simulink model "TBRe19_ECU_Torque_request_TSS_ON"  (R2017b)
settings: Solver=FixedStepDiscrete  StartTime=0.0  StopTime=inf  FixedStep=0.0001  RelTol=1e-3
PostLoadFcn:
  | model_init();
libraries: simulink x17
(part 4 of 6)

== system TBRe19_ECU_Torque_request_TSS_ON/MainTask/Pre_Processing_Layer/Pedal_Box ==
  note: Throttle 20 and Brake 10 are arbitrary values (not rules)
  note: Overall Functionality:
      | - All pedal box sensor values are checked to ensure that they are in the correct voltage range
      | - These sensors are then scaled to be between 0-100 %
      | - APPS Implausibility is performed
      | - Brake pedal implausibility is performed
      | - Thresholds for when brake is considered active, and throttle is considered active are set here (used for RTD and Brake Light activation respectively)
  DAL_In : Inport
  APPS and BP Plausibility : Subsystem
  APPS_Implausibility_Check : Subsystem
  BPPS_Implausibility_Check : Subsystem
  Bus Creator : BusCreator  Inputs=12
  Bus Selector : BusSelector  OutputSignals=DAL_Hardwired.Throttle1_Voltage,DAL_Hardwired.Throttle2_Voltage,DAL_Hardwired.Brake_POT,DAL_Hardwired.Brake1_Pressure,DAL_Hardwired.Brake2_Pressure
  Memory read : S-Function  FunctionName=NsiMem_Read  Parameters=name_var,type_var,size_var,tunable_var  SFunctionDeploymentMode=off  EnableBusSupport=off  mask(Memory read){name_var=Throttle_Active_Threshold, type_var=Unsigned Byte, size_var=1, tunable_var=on}
      mask prompts: name_var "Variable name :"; type_var "Type :"; size_var "Dim of table :"; tunable_var "Is Tunable By USB?"
      mask help: Reads current value of variable memory declared in the configurator block in calibration page.
      mask init:
      | NsiMem_Read_InitializationFcn();
      settings: OpenFcn=NsiMem_Read_OpenFcn();
      mask Help:
      | eval('block=get_param(gcb, ''RTWdata'');')
      | web([docroot '\toolbox\MUXlink\html\blocks/' block.MUXlink_BlockType '.html'])
      mask TypeOptions name_var: Gearing_Ratio | Wheel_Size | Brake1_High | Brake2_High | Throttle1_High | Throttle2_High | Brake1_Low | Brake2_Low | Throttle1_Low | Throttle2_Low | Max_Torque_Std | Max_Torque_Boost | MCU_Ignition | LV_Low_Voltage_Warning | MCUMotor_Temp_Warning | Target_Slip_Ratio | TC_P_Gain | MinTC_Torque | Max_Regen | Throttle_Active_Threshold | Brake_Active_Threshold | INV_Torque_limit | INV_Speed_Limit_Fwd | INV_Speed_limit_Rev | INV_DC_Link_Target | INV_DC_Link_Regen_Imax | INV_DC_Link_Discharge_Imax | INV_Regen_Torque_Limit | INV_Id_Debug | INV_Iq_debug
      mask Callback name_var: NsiMem_Read_ApplyFcn(1);
      mask TypeOptions type_var: Boolean | Signed Byte | Unsigned Byte | Signed Word | Unsigned Word | Signed Double Word | Unsigned Double Word | Single Float | Double Float
      mask Callback type_var: NsiMem_Read_ApplyFcn(2);
      mask Callback size_var: NsiMem_Read_ApplyFcn(3);
      mask Callback tunable_var: NsiMem_Read_ApplyFcn(4);
      mask Display: image(imread('nsi.bmp'));text(0.5, 0.35, 'Throttle_Active_Threshold', 'horizontalAlignment', 'center', 'verticalAlignment', 'base');plot([0.05 0.05 0.05 0.05 0.05 0.05 0.05 0.05 0.05 0.05]);port_label('output', 1, 'Read');
  Memory read1 : S-Function  FunctionName=NsiMem_Read  Parameters=name_var,type_var,size_var,tunable_var  SFunctionDeploymentMode=off  EnableBusSupport=off  mask(Memory read){name_var=Brake_Active_Threshold, type_var=Unsigned Byte, size_var=1, tunable_var=on}
      mask prompts: name_var "Variable name :"; type_var "Type :"; size_var "Dim of table :"; tunable_var "Is Tunable By USB?"
      mask help: Reads current value of variable memory declared in the configurator block in calibration page.
      mask init:
      | NsiMem_Read_InitializationFcn();
      settings: OpenFcn=NsiMem_Read_OpenFcn();
      mask Help:
      | eval('block=get_param(gcb, ''RTWdata'');')
      | web([docroot '\toolbox\MUXlink\html\blocks/' block.MUXlink_BlockType '.html'])
      mask TypeOptions name_var: Gearing_Ratio | Wheel_Size | Brake1_High | Brake2_High | Throttle1_High | Throttle2_High | Brake1_Low | Brake2_Low | Throttle1_Low | Throttle2_Low | Max_Torque_Std | Max_Torque_Boost | MCU_Ignition | LV_Low_Voltage_Warning | MCUMotor_Temp_Warning | Target_Slip_Ratio | TC_P_Gain | MinTC_Torque | Max_Regen | Throttle_Active_Threshold | Brake_Active_Threshold | INV_Torque_limit | INV_Speed_Limit_Fwd | INV_Speed_limit_Rev | INV_DC_Link_Target | INV_DC_Link_Regen_Imax | INV_DC_Link_Discharge_Imax | INV_Regen_Torque_Limit | INV_Id_Debug | INV_Iq_debug
      mask Callback name_var: NsiMem_Read_ApplyFcn(1);
      mask TypeOptions type_var: Boolean | Signed Byte | Unsigned Byte | Signed Word | Unsigned Word | Signed Double Word | Unsigned Double Word | Single Float | Double Float
      mask Callback type_var: NsiMem_Read_ApplyFcn(2);
      mask Callback size_var: NsiMem_Read_ApplyFcn(3);
      mask Callback tunable_var: NsiMem_Read_ApplyFcn(4);
      mask Display: image(imread('nsi.bmp'));text(0.5, 0.35, 'Brake_Active_Threshold', 'horizontalAlignment', 'center', 'verticalAlignment', 'base');plot([0.05 0.05 0.05 0.05 0.05 0.05 0.05 0.05 0.05 0.05]);port_label('output', 1, 'Read');
  Relational Operator : RelationalOperator  OutDataTypeStr=boolean  RndMeth=Simplest
  Relational Operator1 : RelationalOperator  OutDataTypeStr=boolean  RndMeth=Simplest
  Sensor Plausibility : Subsystem
  Terminator : Terminator
  UsbTx1 : S-Function  FunctionName=NsiUsb_Tx  Parameters=signame,resolution,offset,unite  SFunctionDeploymentMode=off  EnableBusSupport=off  mask(MUXlink Usb Tx){signame=Throttle_merge, resolution=1, offset=0, unite=%}
      mask prompts: signame "Signal name ?"; resolution "Resolution ?"; offset "Offset ?"; unite "Unit ?"
      mask help: Transmit a frame on the USB Channel.
      mask init:
      | NsiUsb_Tx_InitializationFcn();
      settings: OpenFcn=NsiUsb_Tx_OpenFcn();
      mask Help:
      | eval('block=get_param(gcb, ''RTWdata'');')
      | web([docroot '\toolbox\MUXlink\html\blocks/' block.MUXlink_BlockType '.html'])
      mask Callback signame: NsiUsb_Tx_ApplyFcn(1);
      mask Callback resolution: NsiUsb_Tx_ApplyFcn(2);
      mask Callback offset: NsiUsb_Tx_ApplyFcn(3);
      mask Callback unite: NsiUsb_Tx_ApplyFcn(4);
      mask Display: image(imread('nsi.bmp'));text(0.5, 0.2, 'USB Tx', 'horizontalAlignment', 'center', 'verticalAlignment', 'base');plot([0.05 0.05 0.05 0.05 0.05 0.05 0.05 0.05 0.05 0.05]);port_label('input',1, 'Throttle_merge');
  Voltage_to_% Conversion : Subsystem
  Pedal_Box_Data : Outport
  wires:
  Bus Creator/1 -> Pedal_Box_Data/1
  DAL_In/1 -> Bus Selector/1
  Voltage_to_% Conversion/1(T1%) -> Bus Creator/2, APPS_Implausibility_Check/1(Throttle1_Per)  "Throttle1_Per"
  Voltage_to_% Conversion/2(T2%) -> Bus Creator/3, APPS_Implausibility_Check/2(Throttle2_Per)  "Throttle2_Per"
  Relational Operator1/1 -> Bus Creator/6  "Throttle_Bool"
  Relational Operator/1 -> Bus Creator/8  "Brake_Bool"
  APPS and BP Plausibility/1(Throttle_%) -> Relational Operator1/1, UsbTx1/1, Bus Creator/5  "Throttle_Percentage"
  APPS and BP Plausibility/2(APPS_BP_Implausibility) -> Bus Creator/7  "APPS_BP_Implausibility"
  APPS_Implausibility_Check/1(APPS_Implausibility) -> Bus Creator/4  "APPS_Implausibility"
  APPS_Implausibility_Check/2(Throttle_%) -> APPS and BP Plausibility/1(Throttle_In)
  Sensor Plausibility/1(Pedal_Sensor_Fail) -> Bus Creator/1  "Pedal_Sensor_Fail"
  Bus Selector/1 -> Sensor Plausibility/1(<Throttle1_Voltage>)  "<Throttle1_Voltage>"
  Bus Selector/2 -> Sensor Plausibility/2(<Throttle2_Voltage>)  "<Throttle2_Voltage>"
  Bus Selector/3 -> Sensor Plausibility/3(<Brake_Voltage>)  "<Brake_POT>"
  Sensor Plausibility/2(TV1_Out) -> Voltage_to_% Conversion/1(Throttle1)
  Sensor Plausibility/3(TV2_Out) -> Voltage_to_% Conversion/2(Throttle2)
  Sensor Plausibility/4(BVPot_Out) -> Voltage_to_% Conversion/3(BrakePOT)
  Bus Selector/4 -> Sensor Plausibility/4(<Brake_Voltage>1)  "<Brake1_Pressure>"
  Bus Selector/5 -> Sensor Plausibility/5(<Brake_Voltage>2)  "<Brake2_Pressure>"
  Sensor Plausibility/5(BV1_Out) -> Voltage_to_% Conversion/4(BrakePress1)
  Sensor Plausibility/6(BV1_Out1) -> Voltage_to_% Conversion/5(BrakePress2)
  BPPS_Implausibility_Check/1(Brake_%) -> Relational Operator/1, Bus Creator/9, APPS and BP Plausibility/2(Brake_%)  "Brake_Percentage"
  BPPS_Implausibility_Check/2(BPPS_Implausibility) -> Bus Creator/10  "BPPS_Implausibility"
  Voltage_to_% Conversion/4(BPr%1) -> Bus Creator/11, BPPS_Implausibility_Check/1(Brake1_Per)  "Brake1_Per"
  Voltage_to_% Conversion/5(BPr%2) -> Bus Creator/12, BPPS_Implausibility_Check/2(Brake2_Per)  "Brake2_Per"
  Voltage_to_% Conversion/3(BPot%) -> Terminator/1  "Brake_%"
  Memory read1/1 -> Relational Operator/2
  Memory read/1 -> Relational Operator1/2

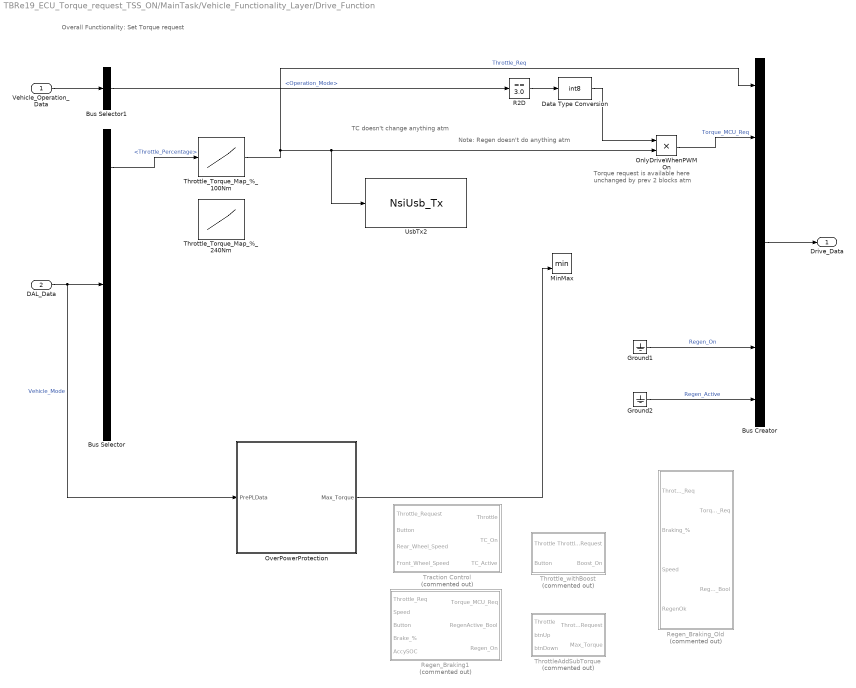
== system TBRe19_ECU_Torque_request_TSS_ON/MainTask/Vehicle_Functionality_Layer/Drive_Function ==
  note: Torque request is available here
      | unchanged by prev 2 blocks atm
  note: TC doesn't change anything atm
  note: Note: Regen doesn't do anything atm
  note: Overall Functionality:
      | Set Torque request
  Vehicle_Operation_Data : Inport
  DAL_Data : Inport  Port=2
  Bus Creator : BusCreator  Inputs=7
  Bus Selector : BusSelector  OutputSignals=Pedal_Box_Data.Throttle_Percentage,DAL_Data.DAL_Hardwired.btnX_Input,DAL_Data.DAL_Hardwired.btnY_Input,DAL_Data.DAL_Hardwired.btnZ_Input
  Bus Selector1 : BusSelector  OutputSignals=Operation_Mode
  Data Type Conversion : DataTypeConversion  OutDataTypeStr=int8
  Ground1 : Ground
  Ground2 : Ground
  MinMax : MinMax  Inputs=2
  OnlyDriveWhenPWMOn : Product  OutDataTypeStr=int16
  OverPowerProtection : Subsystem
  R2D : simulink/Logic and Bit Operations/Compare To Constant  relop===  const=3.0  OutDataTypeStr=boolean
  Regen_Braking1 : Subsystem  Commented=on
  Regen_Braking_Old : Subsystem  Commented=on
  ThrottleAddSubTorque : Subsystem  Commented=on
  Throttle_Torque_Map_%_100Nm : Lookup_n-D  NumberOfTableDimensions=1  BreakpointsForDimension1=[0,25,100]  Table=[0,10,100]  ExtrapMethod=Clip  UseLastTableValue=on  InternalRulePriority=Speed  OutDataTypeStr=int16  RndMeth=Simplest  InputSameDT=on
  Throttle_Torque_Map_%_240Nm : Lookup_n-D  NumberOfTableDimensions=1  BreakpointsForDimension1=[0,25,100]  Table=[0,20,240]  ExtrapMethod=Clip  UseLastTableValue=on  InternalRulePriority=Speed  OutDataTypeStr=int16  RndMeth=Simplest  InputSameDT=on
  Throttle_withBoost : Subsystem  Commented=on
  Traction Control : Subsystem  Commented=on
  UsbTx2 : S-Function  FunctionName=NsiUsb_Tx  Parameters=signame,resolution,offset,unite  SFunctionDeploymentMode=off  EnableBusSupport=off  mask(MUXlink Usb Tx){signame=TorqueRequestInternal, resolution=1, offset=0, unite=Nm}
      mask prompts: signame "Signal name ?"; resolution "Resolution ?"; offset "Offset ?"; unite "Unit ?"
      mask help: Transmit a frame on the USB Channel.
      mask init:
      | NsiUsb_Tx_InitializationFcn();
      settings: OpenFcn=NsiUsb_Tx_OpenFcn();
      mask Help:
      | eval('block=get_param(gcb, ''RTWdata'');')
      | web([docroot '\toolbox\MUXlink\html\blocks/' block.MUXlink_BlockType '.html'])
      mask Callback signame: NsiUsb_Tx_ApplyFcn(1);
      mask Callback resolution: NsiUsb_Tx_ApplyFcn(2);
      mask Callback offset: NsiUsb_Tx_ApplyFcn(3);
      mask Callback unite: NsiUsb_Tx_ApplyFcn(4);
      mask Display: image(imread('nsi.bmp'));text(0.5, 0.2, 'USB Tx', 'horizontalAlignment', 'center', 'verticalAlignment', 'base');plot([0.05 0.05 0.05 0.05 0.05 0.05 0.05 0.05 0.05 0.05]);port_label('input',1, 'TorqueRequestInternal');
  Drive_Data : Outport
  wires:
  Bus Selector1/1 -> R2D/1  "<Operation_Mode>"
  Bus Selector/1 -> Throttle_Torque_Map_%_100Nm/1  "<Throttle_Percentage>"
  R2D/1 -> Data Type Conversion/1
  Vehicle_Operation_Data/1 -> Bus Selector1/1
  DAL_Data/1 -> OverPowerProtection/1(PrePLData), Bus Selector/1  "Vehicle_Mode"
  OnlyDriveWhenPWMOn/1 -> Bus Creator/2  "Torque_MCU_Req"
  Throttle_Torque_Map_%_100Nm/1 -> UsbTx2/1, OnlyDriveWhenPWMOn/2, Bus Creator/1  "Throttle_Req"
  Bus Creator/1 -> Drive_Data/1
  Data Type Conversion/1 -> OnlyDriveWhenPWMOn/1
  Ground1/1 -> Bus Creator/6  "Regen_On"
  OverPowerProtection/1(Max_Torque) -> MinMax/2
  Ground2/1 -> Bus Creator/7  "Regen_Active"

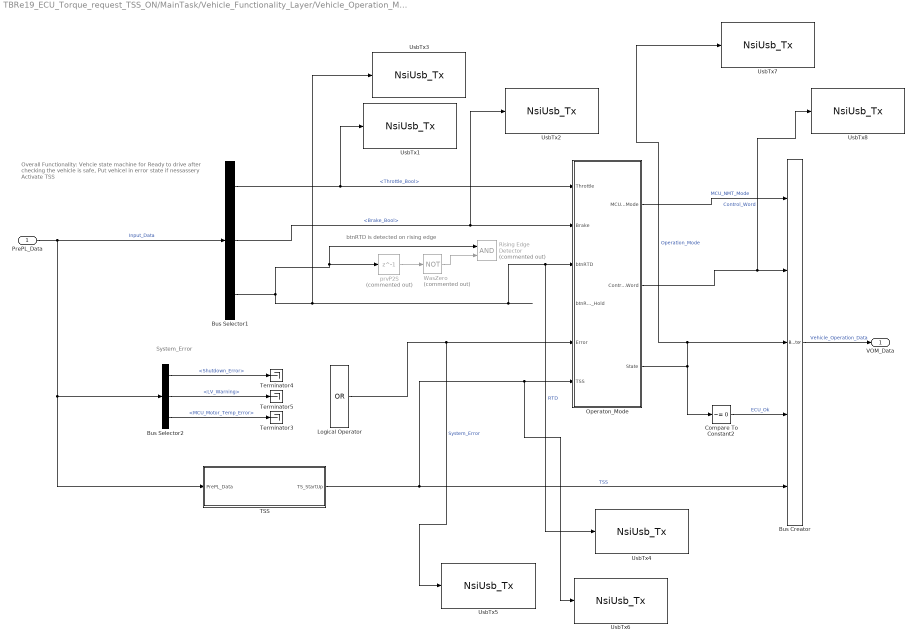
== system TBRe19_ECU_Torque_request_TSS_ON/MainTask/Vehicle_Functionality_Layer/Vehicle_Operation_Mode ==
  note: System_Error
  note: btnRTD is detected on rising edge
  note: Overall Functionality:
      | Vehcie state machine for Ready to drive after checking the vehicle is safe,
      | Put vehicel in error state if nessassery
      | Activate TSS
  PrePL_Data : Inport
  Bus Creator : BusCreator  Inputs=5
  Bus Selector1 : BusSelector  OutputSignals=Pedal_Box_Data.Throttle_Bool,Pedal_Box_Data.Brake_Bool,Buttons.btnRTD
  Bus Selector2 : BusSelector  OutputSignals=DAL_Data.DAL_CAN.DAL_SENSORCAN.Shutdown_Error,LV_Battery.LV_Warning,MCU_Temps_Data.MCU_Motor_Temp_Error
  Compare To Constant2 : simulink/Logic and Bit Operations/Compare To Constant  relop=~=  const=0  OutDataTypeStr=boolean
  Logical Operator : Logic  Operator=OR  Inputs=5  AllPortsSameDT=off  OutDataTypeStr=boolean
  Operaton_Mode : Stateflow chart  TreatAsAtomicUnit=on
  Rising Edge Detector : Logic  Commented=on  AllPortsSameDT=off  OutDataTypeStr=boolean
  TSS : Subsystem
  Terminator3 : Terminator
  Terminator4 : Terminator
  Terminator5 : Terminator
  UsbTx1 : S-Function  FunctionName=NsiUsb_Tx  Parameters=signame,resolution,offset,unite  SFunctionDeploymentMode=off  EnableBusSupport=off  mask(MUXlink Usb Tx){signame=throttle_bool, resolution=1, offset=0, unite=bool}
      mask prompts: signame "Signal name ?"; resolution "Resolution ?"; offset "Offset ?"; unite "Unit ?"
      mask help: Transmit a frame on the USB Channel.
      mask init:
      | NsiUsb_Tx_InitializationFcn();
      settings: OpenFcn=NsiUsb_Tx_OpenFcn();
      mask Help:
      | eval('block=get_param(gcb, ''RTWdata'');')
      | web([docroot '\toolbox\MUXlink\html\blocks/' block.MUXlink_BlockType '.html'])
      mask Callback signame: NsiUsb_Tx_ApplyFcn(1);
      mask Callback resolution: NsiUsb_Tx_ApplyFcn(2);
      mask Callback offset: NsiUsb_Tx_ApplyFcn(3);
      mask Callback unite: NsiUsb_Tx_ApplyFcn(4);
      mask Display: image(imread('nsi.bmp'));text(0.5, 0.2, 'USB Tx', 'horizontalAlignment', 'center', 'verticalAlignment', 'base');plot([0.05 0.05 0.05 0.05 0.05 0.05 0.05 0.05 0.05 0.05]);port_label('input',1, 'throttle_bool');
  UsbTx2 : S-Function  FunctionName=NsiUsb_Tx  Parameters=signame,resolution,offset,unite  SFunctionDeploymentMode=off  EnableBusSupport=off  mask(MUXlink Usb Tx){signame=Brake_bool, resolution=1, offset=0, unite=bool}
      mask prompts: signame "Signal name ?"; resolution "Resolution ?"; offset "Offset ?"; unite "Unit ?"
      mask help: Transmit a frame on the USB Channel.
      mask init:
      | NsiUsb_Tx_InitializationFcn();
      settings: OpenFcn=NsiUsb_Tx_OpenFcn();
      mask Help:
      | eval('block=get_param(gcb, ''RTWdata'');')
      | web([docroot '\toolbox\MUXlink\html\blocks/' block.MUXlink_BlockType '.html'])
      mask Callback signame: NsiUsb_Tx_ApplyFcn(1);
      mask Callback resolution: NsiUsb_Tx_ApplyFcn(2);
      mask Callback offset: NsiUsb_Tx_ApplyFcn(3);
      mask Callback unite: NsiUsb_Tx_ApplyFcn(4);
      mask Display: image(imread('nsi.bmp'));text(0.5, 0.2, 'USB Tx', 'horizontalAlignment', 'center', 'verticalAlignment', 'base');plot([0.05 0.05 0.05 0.05 0.05 0.05 0.05 0.05 0.05 0.05]);port_label('input',1, 'Brake_bool');
  UsbTx3 : S-Function  FunctionName=NsiUsb_Tx  Parameters=signame,resolution,offset,unite  SFunctionDeploymentMode=off  EnableBusSupport=off  mask(MUXlink Usb Tx){signame=rtd_button, resolution=1, offset=0, unite=bool}
      mask prompts: signame "Signal name ?"; resolution "Resolution ?"; offset "Offset ?"; unite "Unit ?"
      mask help: Transmit a frame on the USB Channel.
      mask init:
      | NsiUsb_Tx_InitializationFcn();
      settings: OpenFcn=NsiUsb_Tx_OpenFcn();
      mask Help:
      | eval('block=get_param(gcb, ''RTWdata'');')
      | web([docroot '\toolbox\MUXlink\html\blocks/' block.MUXlink_BlockType '.html'])
      mask Callback signame: NsiUsb_Tx_ApplyFcn(1);
      mask Callback resolution: NsiUsb_Tx_ApplyFcn(2);
      mask Callback offset: NsiUsb_Tx_ApplyFcn(3);
      mask Callback unite: NsiUsb_Tx_ApplyFcn(4);
      mask Display: image(imread('nsi.bmp'));text(0.5, 0.2, 'USB Tx', 'horizontalAlignment', 'center', 'verticalAlignment', 'base');plot([0.05 0.05 0.05 0.05 0.05 0.05 0.05 0.05 0.05 0.05]);port_label('input',1, 'rtd_button');
  UsbTx4 : S-Function  FunctionName=NsiUsb_Tx  Parameters=signame,resolution,offset,unite  SFunctionDeploymentMode=off  EnableBusSupport=off  mask(MUXlink Usb Tx){signame=rtd_button_State_in, resolution=1, offset=0, unite=bool}
      mask prompts: signame "Signal name ?"; resolution "Resolution ?"; offset "Offset ?"; unite "Unit ?"
      mask help: Transmit a frame on the USB Channel.
      mask init:
      | NsiUsb_Tx_InitializationFcn();
      settings: OpenFcn=NsiUsb_Tx_OpenFcn();
      mask Help:
      | eval('block=get_param(gcb, ''RTWdata'');')
      | web([docroot '\toolbox\MUXlink\html\blocks/' block.MUXlink_BlockType '.html'])
      mask Callback signame: NsiUsb_Tx_ApplyFcn(1);
      mask Callback resolution: NsiUsb_Tx_ApplyFcn(2);
      mask Callback offset: NsiUsb_Tx_ApplyFcn(3);
      mask Callback unite: NsiUsb_Tx_ApplyFcn(4);
      mask Display: image(imread('nsi.bmp'));text(0.5, 0.2, 'USB Tx', 'horizontalAlignment', 'center', 'verticalAlignment', 'base');plot([0.05 0.05 0.05 0.05 0.05 0.05 0.05 0.05 0.05 0.05]);port_label('input',1, 'rtd_button_State_in');
  UsbTx5 : S-Function  FunctionName=NsiUsb_Tx  Parameters=signame,resolution,offset,unite  SFunctionDeploymentMode=off  EnableBusSupport=off  mask(MUXlink Usb Tx){signame=rtd_error, resolution=1, offset=0, unite=bool}
      mask prompts: signame "Signal name ?"; resolution "Resolution ?"; offset "Offset ?"; unite "Unit ?"
      mask help: Transmit a frame on the USB Channel.
      mask init:
      | NsiUsb_Tx_InitializationFcn();
      settings: OpenFcn=NsiUsb_Tx_OpenFcn();
      mask Help:
      | eval('block=get_param(gcb, ''RTWdata'');')
      | web([docroot '\toolbox\MUXlink\html\blocks/' block.MUXlink_BlockType '.html'])
      mask Callback signame: NsiUsb_Tx_ApplyFcn(1);
      mask Callback resolution: NsiUsb_Tx_ApplyFcn(2);
      mask Callback offset: NsiUsb_Tx_ApplyFcn(3);
      mask Callback unite: NsiUsb_Tx_ApplyFcn(4);
      mask Display: image(imread('nsi.bmp'));text(0.5, 0.2, 'USB Tx', 'horizontalAlignment', 'center', 'verticalAlignment', 'base');plot([0.05 0.05 0.05 0.05 0.05 0.05 0.05 0.05 0.05 0.05]);port_label('input',1, 'rtd_error');
  UsbTx6 : S-Function  FunctionName=NsiUsb_Tx  Parameters=signame,resolution,offset,unite  SFunctionDeploymentMode=off  EnableBusSupport=off  mask(MUXlink Usb Tx){signame=rtd_tss, resolution=1, offset=0, unite=bool}
      mask prompts: signame "Signal name ?"; resolution "Resolution ?"; offset "Offset ?"; unite "Unit ?"
      mask help: Transmit a frame on the USB Channel.
      mask init:
      | NsiUsb_Tx_InitializationFcn();
      settings: OpenFcn=NsiUsb_Tx_OpenFcn();
      mask Help:
      | eval('block=get_param(gcb, ''RTWdata'');')
      | web([docroot '\toolbox\MUXlink\html\blocks/' block.MUXlink_BlockType '.html'])
      mask Callback signame: NsiUsb_Tx_ApplyFcn(1);
      mask Callback resolution: NsiUsb_Tx_ApplyFcn(2);
      mask Callback offset: NsiUsb_Tx_ApplyFcn(3);
      mask Callback unite: NsiUsb_Tx_ApplyFcn(4);
      mask Display: image(imread('nsi.bmp'));text(0.5, 0.2, 'USB Tx', 'horizontalAlignment', 'center', 'verticalAlignment', 'base');plot([0.05 0.05 0.05 0.05 0.05 0.05 0.05 0.05 0.05 0.05]);port_label('input',1, 'rtd_tss');
  UsbTx7 : S-Function  FunctionName=NsiUsb_Tx  Parameters=signame,resolution,offset,unite  SFunctionDeploymentMode=off  EnableBusSupport=off  mask(MUXlink Usb Tx){signame=RTD_state, resolution=1, offset=0, unite=bool}
      mask prompts: signame "Signal name ?"; resolution "Resolution ?"; offset "Offset ?"; unite "Unit ?"
      mask help: Transmit a frame on the USB Channel.
      mask init:
      | NsiUsb_Tx_InitializationFcn();
      settings: OpenFcn=NsiUsb_Tx_OpenFcn();
      mask Help:
      | eval('block=get_param(gcb, ''RTWdata'');')
      | web([docroot '\toolbox\MUXlink\html\blocks/' block.MUXlink_BlockType '.html'])
      mask Callback signame: NsiUsb_Tx_ApplyFcn(1);
      mask Callback resolution: NsiUsb_Tx_ApplyFcn(2);
      mask Callback offset: NsiUsb_Tx_ApplyFcn(3);
      mask Callback unite: NsiUsb_Tx_ApplyFcn(4);
      mask Display: image(imread('nsi.bmp'));text(0.5, 0.2, 'USB Tx', 'horizontalAlignment', 'center', 'verticalAlignment', 'base');plot([0.05 0.05 0.05 0.05 0.05 0.05 0.05 0.05 0.05 0.05]);port_label('input',1, 'RTD_state');
  UsbTx8 : S-Function  FunctionName=NsiUsb_Tx  Parameters=signame,resolution,offset,unite  SFunctionDeploymentMode=off  EnableBusSupport=off  mask(MUXlink Usb Tx){signame=INV_control_word, resolution=1, offset=0, unite=bool}
      mask prompts: signame "Signal name ?"; resolution "Resolution ?"; offset "Offset ?"; unite "Unit ?"
      mask help: Transmit a frame on the USB Channel.
      mask init:
      | NsiUsb_Tx_InitializationFcn();
      settings: OpenFcn=NsiUsb_Tx_OpenFcn();
      mask Help:
      | eval('block=get_param(gcb, ''RTWdata'');')
      | web([docroot '\toolbox\MUXlink\html\blocks/' block.MUXlink_BlockType '.html'])
      mask Callback signame: NsiUsb_Tx_ApplyFcn(1);
      mask Callback resolution: NsiUsb_Tx_ApplyFcn(2);
      mask Callback offset: NsiUsb_Tx_ApplyFcn(3);
      mask Callback unite: NsiUsb_Tx_ApplyFcn(4);
      mask Display: image(imread('nsi.bmp'));text(0.5, 0.2, 'USB Tx', 'horizontalAlignment', 'center', 'verticalAlignment', 'base');plot([0.05 0.05 0.05 0.05 0.05 0.05 0.05 0.05 0.05 0.05]);port_label('input',1, 'INV_control_word');
  WasZero : Logic  Commented=on  Operator=NOT  AllPortsSameDT=off  OutDataTypeStr=boolean
  prvP2S : Delay  Commented=on  DelayLength=1  InitialCondition=0
  VOM_Data : Outport
  wires:
  Bus Selector1/2 -> UsbTx2/1, Operaton_Mode/2(Brake)  "<Brake_Bool>"
  Compare To Constant2/1 -> Bus Creator/4  "ECU_Ok"
  Operaton_Mode/2(Control_Word) -> UsbTx8/1, Bus Creator/2  "Control_Word"
  Operaton_Mode/1(MCU_NMT_Mode) -> Bus Creator/1  "MCU_NMT_Mode"
  Operaton_Mode/3(State) -> Bus Creator/3, UsbTx7/1, Compare To Constant2/1  "Operation_Mode"
  Bus Creator/1 -> VOM_Data/1  "Vehicle_Operation_Data"
  Bus Selector1/1 -> UsbTx1/1, Operaton_Mode/1(Throttle)  "<Throttle_Bool>"
  TSS/1(TS_StartUp) -> UsbTx6/1, Operaton_Mode/6(TSS), Bus Creator/5  "TSS"
  WasZero/1 -> Rising Edge Detector/2
  prvP2S/1 -> WasZero/1
  Bus Selector1/3 -> prvP2S/1, Rising Edge Detector/1, UsbTx3/1, UsbTx4/1, Operaton_Mode/3(btnRTD)  "RTD"
  Bus Selector2/3 -> Terminator3/1  "<MCU_Motor_Temp_Error>"
  Bus Selector2/2 -> Terminator5/1  "<LV_Warning>"
  Bus Selector2/1 -> Terminator4/1  "<Shutdown_Error>"
  Logical Operator/1 -> UsbTx5/1, Operaton_Mode/5(Error)  "System_Error"
  PrePL_Data/1 -> Bus Selector2/1, TSS/1(PrePL_Data), Bus Selector1/1  "Input_Data"

== system TBRe19_ECU_Torque_request_TSS_ON/MainTask/Comms_And_Data_Acquisition_Layer/Hardwired_Inputs_2019/AIRs ==
  DigitalInput : S-Function  FunctionName=NsiIo_DigitalInput  Parameters=channel,is_trigger,typeof_trigger,is_wakeup,wakeup_level  SFunctionDeploymentMode=off  EnableBusSupport=off  mask(MUXlink I/O Digital Input){channel=1, is_trigger=off, typeof_trigger=Either, is_wakeup=off, wakeup_level=Low level}
      mask prompts: channel "Channel ?"; is_trigger "Trigger ?"; typeof_trigger "Type of Trigger ?"; is_wakeup "Wake-up ?"; wakeup_level "Wake-up level ?"
      mask help: Read digital input from I/O channel.
      mask init:
      | NsiIo_DigitalInput_InitializationFcn();
      settings: OpenFcn=NsiIo_DigitalInput_OpenFcn();
      mask Help:
      | eval('block=get_param(gcb, ''RTWdata'');')
      | web([docroot '\toolbox\MUXlink\html\blocks/' block.MUXlink_BlockType '.html'])
      mask Callback channel: NsiIo_DigitalInput_ApplyFcn(1);
      mask Callback is_trigger: NsiIo_DigitalInput_ApplyFcn(2);
      mask TypeOptions typeof_trigger: Rising | Falling | Either
      mask Callback typeof_trigger: NsiIo_DigitalInput_ApplyFcn(3);
      mask Callback is_wakeup: NsiIo_DigitalInput_ApplyFcn(4);
      mask TypeOptions wakeup_level: Low level | High level
      mask Callback wakeup_level: NsiIo_DigitalInput_ApplyFcn(5);
      mask Display: image(imread('nsi.bmp'));text(0.5, 0.2, 'DigitalInput_1', 'horizontalAlignment', 'center', 'verticalAlignment', 'base');plot([0.05 0.05 0.05 0.05 0.05 0.05 0.05 0.05 0.05 0.05]);port_label('output', 1, 'Ground : A1');
  DigitalInput5 : S-Function  FunctionName=NsiIo_DigitalInput  Parameters=channel,is_trigger,typeof_trigger,is_wakeup,wakeup_level  SFunctionDeploymentMode=off  EnableBusSupport=off  mask(MUXlink I/O Digital Input){channel=2, is_trigger=off, typeof_trigger=Either, is_wakeup=off, wakeup_level=Low level}
      mask prompts: channel "Channel ?"; is_trigger "Trigger ?"; typeof_trigger "Type of Trigger ?"; is_wakeup "Wake-up ?"; wakeup_level "Wake-up level ?"
      mask help: Read digital input from I/O channel.
      mask init:
      | NsiIo_DigitalInput_InitializationFcn();
      settings: OpenFcn=NsiIo_DigitalInput_OpenFcn();
      mask Help:
      | eval('block=get_param(gcb, ''RTWdata'');')
      | web([docroot '\toolbox\MUXlink\html\blocks/' block.MUXlink_BlockType '.html'])
      mask Callback channel: NsiIo_DigitalInput_ApplyFcn(1);
      mask Callback is_trigger: NsiIo_DigitalInput_ApplyFcn(2);
      mask TypeOptions typeof_trigger: Rising | Falling | Either
      mask Callback typeof_trigger: NsiIo_DigitalInput_ApplyFcn(3);
      mask Callback is_wakeup: NsiIo_DigitalInput_ApplyFcn(4);
      mask TypeOptions wakeup_level: Low level | High level
      mask Callback wakeup_level: NsiIo_DigitalInput_ApplyFcn(5);
      mask Display: image(imread('nsi.bmp'));text(0.5, 0.2, 'DigitalInput_2', 'horizontalAlignment', 'center', 'verticalAlignment', 'base');plot([0.05 0.05 0.05 0.05 0.05 0.05 0.05 0.05 0.05 0.05]);port_label('output', 1, 'Ground : A2');
  UsbTx1 : S-Function  FunctionName=NsiUsb_Tx  Parameters=signame,resolution,offset,unite  SFunctionDeploymentMode=off  EnableBusSupport=off  mask(MUXlink Usb Tx){signame=AIRLow, resolution=1, offset=0, unite=Bool}
      mask prompts: signame "Signal name ?"; resolution "Resolution ?"; offset "Offset ?"; unite "Unit ?"
      mask help: Transmit a frame on the USB Channel.
      mask init:
      | NsiUsb_Tx_InitializationFcn();
      settings: OpenFcn=NsiUsb_Tx_OpenFcn();
      mask Help:
      | eval('block=get_param(gcb, ''RTWdata'');')
      | web([docroot '\toolbox\MUXlink\html\blocks/' block.MUXlink_BlockType '.html'])
      mask Callback signame: NsiUsb_Tx_ApplyFcn(1);
      mask Callback resolution: NsiUsb_Tx_ApplyFcn(2);
      mask Callback offset: NsiUsb_Tx_ApplyFcn(3);
      mask Callback unite: NsiUsb_Tx_ApplyFcn(4);
      mask Display: image(imread('nsi.bmp'));text(0.5, 0.2, 'USB Tx', 'horizontalAlignment', 'center', 'verticalAlignment', 'base');plot([0.05 0.05 0.05 0.05 0.05 0.05 0.05 0.05 0.05 0.05]);port_label('input',1, 'AIRLow');
  UsbTx2 : S-Function  FunctionName=NsiUsb_Tx  Parameters=signame,resolution,offset,unite  SFunctionDeploymentMode=off  EnableBusSupport=off  mask(MUXlink Usb Tx){signame=AIRHigh, resolution=1, offset=0, unite=Bool}
      mask prompts: signame "Signal name ?"; resolution "Resolution ?"; offset "Offset ?"; unite "Unit ?"
      mask help: Transmit a frame on the USB Channel.
      mask init:
      | NsiUsb_Tx_InitializationFcn();
      settings: OpenFcn=NsiUsb_Tx_OpenFcn();
      mask Help:
      | eval('block=get_param(gcb, ''RTWdata'');')
      | web([docroot '\toolbox\MUXlink\html\blocks/' block.MUXlink_BlockType '.html'])
      mask Callback signame: NsiUsb_Tx_ApplyFcn(1);
      mask Callback resolution: NsiUsb_Tx_ApplyFcn(2);
      mask Callback offset: NsiUsb_Tx_ApplyFcn(3);
      mask Callback unite: NsiUsb_Tx_ApplyFcn(4);
      mask Display: image(imread('nsi.bmp'));text(0.5, 0.2, 'USB Tx', 'horizontalAlignment', 'center', 'verticalAlignment', 'base');plot([0.05 0.05 0.05 0.05 0.05 0.05 0.05 0.05 0.05 0.05]);port_label('input',1, 'AIRHigh');
  AIRLow : Outport
  AIRHigh : Outport  Port=2
  wires:
  DigitalInput/1 -> UsbTx1/1, AIRLow/1  "AIRLow"
  DigitalInput5/1 -> UsbTx2/1, AIRHigh/1  "AIRHigh"

== system TBRe19_ECU_Torque_request_TSS_ON/MainTask/Comms_And_Data_Acquisition_Layer/Hardwired_Inputs_2019/BMS ==
  DigitalInput1 : S-Function  FunctionName=NsiIo_DigitalInput  Parameters=channel,is_trigger,typeof_trigger,is_wakeup,wakeup_level  SFunctionDeploymentMode=off  EnableBusSupport=off  mask(MUXlink I/O Digital Input){channel=16, is_trigger=off, typeof_trigger=Either, is_wakeup=off, wakeup_level=Low level}
      mask prompts: channel "Channel ?"; is_trigger "Trigger ?"; typeof_trigger "Type of Trigger ?"; is_wakeup "Wake-up ?"; wakeup_level "Wake-up level ?"
      mask help: Read digital input from I/O channel.
      mask init:
      | NsiIo_DigitalInput_InitializationFcn();
      settings: OpenFcn=NsiIo_DigitalInput_OpenFcn();
      mask Help:
      | eval('block=get_param(gcb, ''RTWdata'');')
      | web([docroot '\toolbox\MUXlink\html\blocks/' block.MUXlink_BlockType '.html'])
      mask Callback channel: NsiIo_DigitalInput_ApplyFcn(1);
      mask Callback is_trigger: NsiIo_DigitalInput_ApplyFcn(2);
      mask TypeOptions typeof_trigger: Rising | Falling | Either
      mask Callback typeof_trigger: NsiIo_DigitalInput_ApplyFcn(3);
      mask Callback is_wakeup: NsiIo_DigitalInput_ApplyFcn(4);
      mask TypeOptions wakeup_level: Low level | High level
      mask Callback wakeup_level: NsiIo_DigitalInput_ApplyFcn(5);
      mask Display: image(imread('nsi.bmp'));text(0.5, 0.2, 'DigitalInput_16', 'horizontalAlignment', 'center', 'verticalAlignment', 'base');plot([0.05 0.05 0.05 0.05 0.05 0.05 0.05 0.05 0.05 0.05]);port_label('output', 1, 'Battery : H2');
  DigitalInput2 : S-Function  FunctionName=NsiIo_DigitalInput  Parameters=channel,is_trigger,typeof_trigger,is_wakeup,wakeup_level  SFunctionDeploymentMode=off  EnableBusSupport=off  mask(MUXlink I/O Digital Input){channel=17, is_trigger=off, typeof_trigger=Either, is_wakeup=off, wakeup_level=Low level}
      mask prompts: channel "Channel ?"; is_trigger "Trigger ?"; typeof_trigger "Type of Trigger ?"; is_wakeup "Wake-up ?"; wakeup_level "Wake-up level ?"
      mask help: Read digital input from I/O channel.
      mask init:
      | NsiIo_DigitalInput_InitializationFcn();
      settings: OpenFcn=NsiIo_DigitalInput_OpenFcn();
      mask Help:
      | eval('block=get_param(gcb, ''RTWdata'');')
      | web([docroot '\toolbox\MUXlink\html\blocks/' block.MUXlink_BlockType '.html'])
      mask Callback channel: NsiIo_DigitalInput_ApplyFcn(1);
      mask Callback is_trigger: NsiIo_DigitalInput_ApplyFcn(2);
      mask TypeOptions typeof_trigger: Rising | Falling | Either
      mask Callback typeof_trigger: NsiIo_DigitalInput_ApplyFcn(3);
      mask Callback is_wakeup: NsiIo_DigitalInput_ApplyFcn(4);
      mask TypeOptions wakeup_level: Low level | High level
      mask Callback wakeup_level: NsiIo_DigitalInput_ApplyFcn(5);
      mask Display: image(imread('nsi.bmp'));text(0.5, 0.2, 'DigitalInput_17', 'horizontalAlignment', 'center', 'verticalAlignment', 'base');plot([0.05 0.05 0.05 0.05 0.05 0.05 0.05 0.05 0.05 0.05]);port_label('output', 1, 'Battery : H3');
  DigitalInput6 : S-Function  FunctionName=NsiIo_DigitalInput  Parameters=channel,is_trigger,typeof_trigger,is_wakeup,wakeup_level  SFunctionDeploymentMode=off  EnableBusSupport=off  mask(MUXlink I/O Digital Input){channel=18, is_trigger=off, typeof_trigger=Either, is_wakeup=off, wakeup_level=Low level}
      mask prompts: channel "Channel ?"; is_trigger "Trigger ?"; typeof_trigger "Type of Trigger ?"; is_wakeup "Wake-up ?"; wakeup_level "Wake-up level ?"
      mask help: Read digital input from I/O channel.
      mask init:
      | NsiIo_DigitalInput_InitializationFcn();
      settings: OpenFcn=NsiIo_DigitalInput_OpenFcn();
      mask Help:
      | eval('block=get_param(gcb, ''RTWdata'');')
      | web([docroot '\toolbox\MUXlink\html\blocks/' block.MUXlink_BlockType '.html'])
      mask Callback channel: NsiIo_DigitalInput_ApplyFcn(1);
      mask Callback is_trigger: NsiIo_DigitalInput_ApplyFcn(2);
      mask TypeOptions typeof_trigger: Rising | Falling | Either
      mask Callback typeof_trigger: NsiIo_DigitalInput_ApplyFcn(3);
      mask Callback is_wakeup: NsiIo_DigitalInput_ApplyFcn(4);
      mask TypeOptions wakeup_level: Low level | High level
      mask Callback wakeup_level: NsiIo_DigitalInput_ApplyFcn(5);
      mask Display: image(imread('nsi.bmp'));text(0.5, 0.2, 'DigitalInput_18', 'horizontalAlignment', 'center', 'verticalAlignment', 'base');plot([0.05 0.05 0.05 0.05 0.05 0.05 0.05 0.05 0.05 0.05]);port_label('output', 1, 'Battery : H4');
  BMS_Multi1 : Outport
  BMS_Multi2 : Outport  Port=2
  BMS_ChargeEnable : Outport  Port=3
  wires:
  DigitalInput6/1 -> BMS_Multi1/1  "BMS_Multi1"
  DigitalInput2/1 -> BMS_ChargeEnable/1  "BMS_ChargeEnable"
  DigitalInput1/1 -> BMS_Multi2/1  "BMS_Multi2"

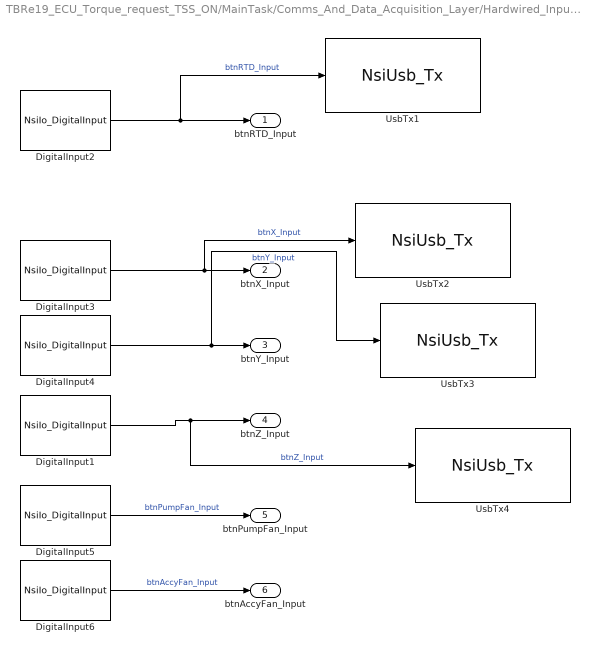
== system TBRe19_ECU_Torque_request_TSS_ON/MainTask/Comms_And_Data_Acquisition_Layer/Hardwired_Inputs_2019/Buttons ==
  DigitalInput1 : S-Function  FunctionName=NsiIo_DigitalInput  Parameters=channel,is_trigger,typeof_trigger,is_wakeup,wakeup_level  SFunctionDeploymentMode=off  EnableBusSupport=off  mask(MUXlink I/O Digital Input){channel=14, is_trigger=off, typeof_trigger=Either, is_wakeup=off, wakeup_level=Low level}
      mask prompts: channel "Channel ?"; is_trigger "Trigger ?"; typeof_trigger "Type of Trigger ?"; is_wakeup "Wake-up ?"; wakeup_level "Wake-up level ?"
      mask help: Read digital input from I/O channel.
      mask init:
      | NsiIo_DigitalInput_InitializationFcn();
      settings: OpenFcn=NsiIo_DigitalInput_OpenFcn();
      mask Help:
      | eval('block=get_param(gcb, ''RTWdata'');')
      | web([docroot '\toolbox\MUXlink\html\blocks/' block.MUXlink_BlockType '.html'])
      mask Callback channel: NsiIo_DigitalInput_ApplyFcn(1);
      mask Callback is_trigger: NsiIo_DigitalInput_ApplyFcn(2);
      mask TypeOptions typeof_trigger: Rising | Falling | Either
      mask Callback typeof_trigger: NsiIo_DigitalInput_ApplyFcn(3);
      mask Callback is_wakeup: NsiIo_DigitalInput_ApplyFcn(4);
      mask TypeOptions wakeup_level: Low level | High level
      mask Callback wakeup_level: NsiIo_DigitalInput_ApplyFcn(5);
      mask Display: image(imread('nsi.bmp'));text(0.5, 0.2, 'DigitalInput_14', 'horizontalAlignment', 'center', 'verticalAlignment', 'base');plot([0.05 0.05 0.05 0.05 0.05 0.05 0.05 0.05 0.05 0.05]);port_label('output', 1, 'Battery : G4');
  DigitalInput2 : S-Function  FunctionName=NsiIo_DigitalInput  Parameters=channel,is_trigger,typeof_trigger,is_wakeup,wakeup_level  SFunctionDeploymentMode=off  EnableBusSupport=off  mask(MUXlink I/O Digital Input){channel=11, is_trigger=off, typeof_trigger=Either, is_wakeup=off, wakeup_level=Low level}
      mask prompts: channel "Channel ?"; is_trigger "Trigger ?"; typeof_trigger "Type of Trigger ?"; is_wakeup "Wake-up ?"; wakeup_level "Wake-up level ?"
      mask help: Read digital input from I/O channel.
      mask init:
      | NsiIo_DigitalInput_InitializationFcn();
      settings: OpenFcn=NsiIo_DigitalInput_OpenFcn();
      mask Help:
      | eval('block=get_param(gcb, ''RTWdata'');')
      | web([docroot '\toolbox\MUXlink\html\blocks/' block.MUXlink_BlockType '.html'])
      mask Callback channel: NsiIo_DigitalInput_ApplyFcn(1);
      mask Callback is_trigger: NsiIo_DigitalInput_ApplyFcn(2);
      mask TypeOptions typeof_trigger: Rising | Falling | Either
      mask Callback typeof_trigger: NsiIo_DigitalInput_ApplyFcn(3);
      mask Callback is_wakeup: NsiIo_DigitalInput_ApplyFcn(4);
      mask TypeOptions wakeup_level: Low level | High level
      mask Callback wakeup_level: NsiIo_DigitalInput_ApplyFcn(5);
      mask Display: image(imread('nsi.bmp'));text(0.5, 0.2, 'DigitalInput_11', 'horizontalAlignment', 'center', 'verticalAlignment', 'base');plot([0.05 0.05 0.05 0.05 0.05 0.05 0.05 0.05 0.05 0.05]);port_label('output', 1, 'Battery : G1');
  DigitalInput3 : S-Function  FunctionName=NsiIo_DigitalInput  Parameters=channel,is_trigger,typeof_trigger,is_wakeup,wakeup_level  SFunctionDeploymentMode=off  EnableBusSupport=off  mask(MUXlink I/O Digital Input){channel=12, is_trigger=off, typeof_trigger=Either, is_wakeup=off, wakeup_level=Low level}
      mask prompts: channel "Channel ?"; is_trigger "Trigger ?"; typeof_trigger "Type of Trigger ?"; is_wakeup "Wake-up ?"; wakeup_level "Wake-up level ?"
      mask help: Read digital input from I/O channel.
      mask init:
      | NsiIo_DigitalInput_InitializationFcn();
      settings: OpenFcn=NsiIo_DigitalInput_OpenFcn();
      mask Help:
      | eval('block=get_param(gcb, ''RTWdata'');')
      | web([docroot '\toolbox\MUXlink\html\blocks/' block.MUXlink_BlockType '.html'])
      mask Callback channel: NsiIo_DigitalInput_ApplyFcn(1);
      mask Callback is_trigger: NsiIo_DigitalInput_ApplyFcn(2);
      mask TypeOptions typeof_trigger: Rising | Falling | Either
      mask Callback typeof_trigger: NsiIo_DigitalInput_ApplyFcn(3);
      mask Callback is_wakeup: NsiIo_DigitalInput_ApplyFcn(4);
      mask TypeOptions wakeup_level: Low level | High level
      mask Callback wakeup_level: NsiIo_DigitalInput_ApplyFcn(5);
      mask Display: image(imread('nsi.bmp'));text(0.5, 0.2, 'DigitalInput_12', 'horizontalAlignment', 'center', 'verticalAlignment', 'base');plot([0.05 0.05 0.05 0.05 0.05 0.05 0.05 0.05 0.05 0.05]);port_label('output', 1, 'Battery : G2');
  DigitalInput4 : S-Function  FunctionName=NsiIo_DigitalInput  Parameters=channel,is_trigger,typeof_trigger,is_wakeup,wakeup_level  SFunctionDeploymentMode=off  EnableBusSupport=off  mask(MUXlink I/O Digital Input){channel=13, is_trigger=off, typeof_trigger=Either, is_wakeup=off, wakeup_level=Low level}
      mask prompts: channel "Channel ?"; is_trigger "Trigger ?"; typeof_trigger "Type of Trigger ?"; is_wakeup "Wake-up ?"; wakeup_level "Wake-up level ?"
      mask help: Read digital input from I/O channel.
      mask init:
      | NsiIo_DigitalInput_InitializationFcn();
      settings: OpenFcn=NsiIo_DigitalInput_OpenFcn();
      mask Help:
      | eval('block=get_param(gcb, ''RTWdata'');')
      | web([docroot '\toolbox\MUXlink\html\blocks/' block.MUXlink_BlockType '.html'])
      mask Callback channel: NsiIo_DigitalInput_ApplyFcn(1);
      mask Callback is_trigger: NsiIo_DigitalInput_ApplyFcn(2);
      mask TypeOptions typeof_trigger: Rising | Falling | Either
      mask Callback typeof_trigger: NsiIo_DigitalInput_ApplyFcn(3);
      mask Callback is_wakeup: NsiIo_DigitalInput_ApplyFcn(4);
      mask TypeOptions wakeup_level: Low level | High level
      mask Callback wakeup_level: NsiIo_DigitalInput_ApplyFcn(5);
      mask Display: image(imread('nsi.bmp'));text(0.5, 0.2, 'DigitalInput_13', 'horizontalAlignment', 'center', 'verticalAlignment', 'base');plot([0.05 0.05 0.05 0.05 0.05 0.05 0.05 0.05 0.05 0.05]);port_label('output', 1, 'Battery : G3');
  DigitalInput5 : S-Function  FunctionName=NsiIo_DigitalInput  Parameters=channel,is_trigger,typeof_trigger,is_wakeup,wakeup_level  SFunctionDeploymentMode=off  EnableBusSupport=off  mask(MUXlink I/O Digital Input){channel=9, is_trigger=off, typeof_trigger=Either, is_wakeup=off, wakeup_level=Low level}
      mask prompts: channel "Channel ?"; is_trigger "Trigger ?"; typeof_trigger "Type of Trigger ?"; is_wakeup "Wake-up ?"; wakeup_level "Wake-up level ?"
      mask help: Read digital input from I/O channel.
      mask init:
      | NsiIo_DigitalInput_InitializationFcn();
      settings: OpenFcn=NsiIo_DigitalInput_OpenFcn();
      mask Help:
      | eval('block=get_param(gcb, ''RTWdata'');')
      | web([docroot '\toolbox\MUXlink\html\blocks/' block.MUXlink_BlockType '.html'])
      mask Callback channel: NsiIo_DigitalInput_ApplyFcn(1);
      mask Callback is_trigger: NsiIo_DigitalInput_ApplyFcn(2);
      mask TypeOptions typeof_trigger: Rising | Falling | Either
      mask Callback typeof_trigger: NsiIo_DigitalInput_ApplyFcn(3);
      mask Callback is_wakeup: NsiIo_DigitalInput_ApplyFcn(4);
      mask TypeOptions wakeup_level: Low level | High level
      mask Callback wakeup_level: NsiIo_DigitalInput_ApplyFcn(5);
      mask Display: image(imread('nsi.bmp'));text(0.5, 0.2, 'DigitalInput_9', 'horizontalAlignment', 'center', 'verticalAlignment', 'base');plot([0.05 0.05 0.05 0.05 0.05 0.05 0.05 0.05 0.05 0.05]);port_label('output', 1, 'Ground : C1');
  DigitalInput6 : S-Function  FunctionName=NsiIo_DigitalInput  Parameters=channel,is_trigger,typeof_trigger,is_wakeup,wakeup_level  SFunctionDeploymentMode=off  EnableBusSupport=off  mask(MUXlink I/O Digital Input){channel=10, is_trigger=off, typeof_trigger=Either, is_wakeup=off, wakeup_level=Low level}
      mask prompts: channel "Channel ?"; is_trigger "Trigger ?"; typeof_trigger "Type of Trigger ?"; is_wakeup "Wake-up ?"; wakeup_level "Wake-up level ?"
      mask help: Read digital input from I/O channel.
      mask init:
      | NsiIo_DigitalInput_InitializationFcn();
      settings: OpenFcn=NsiIo_DigitalInput_OpenFcn();
      mask Help:
      | eval('block=get_param(gcb, ''RTWdata'');')
      | web([docroot '\toolbox\MUXlink\html\blocks/' block.MUXlink_BlockType '.html'])
      mask Callback channel: NsiIo_DigitalInput_ApplyFcn(1);
      mask Callback is_trigger: NsiIo_DigitalInput_ApplyFcn(2);
      mask TypeOptions typeof_trigger: Rising | Falling | Either
      mask Callback typeof_trigger: NsiIo_DigitalInput_ApplyFcn(3);
      mask Callback is_wakeup: NsiIo_DigitalInput_ApplyFcn(4);
      mask TypeOptions wakeup_level: Low level | High level
      mask Callback wakeup_level: NsiIo_DigitalInput_ApplyFcn(5);
      mask Display: image(imread('nsi.bmp'));text(0.5, 0.2, 'DigitalInput_10', 'horizontalAlignment', 'center', 'verticalAlignment', 'base');plot([0.05 0.05 0.05 0.05 0.05 0.05 0.05 0.05 0.05 0.05]);port_label('output', 1, 'Ground : C2');
  UsbTx1 : S-Function  FunctionName=NsiUsb_Tx  Parameters=signame,resolution,offset,unite  SFunctionDeploymentMode=off  EnableBusSupport=off  mask(MUXlink Usb Tx){signame=rtd, resolution=1, offset=0, unite=km/h}
      mask prompts: signame "Signal name ?"; resolution "Resolution ?"; offset "Offset ?"; unite "Unit ?"
      mask help: Transmit a frame on the USB Channel.
      mask init:
      | NsiUsb_Tx_InitializationFcn();
      settings: OpenFcn=NsiUsb_Tx_OpenFcn();
      mask Help:
      | eval('block=get_param(gcb, ''RTWdata'');')
      | web([docroot '\toolbox\MUXlink\html\blocks/' block.MUXlink_BlockType '.html'])
      mask Callback signame: NsiUsb_Tx_ApplyFcn(1);
      mask Callback resolution: NsiUsb_Tx_ApplyFcn(2);
      mask Callback offset: NsiUsb_Tx_ApplyFcn(3);
      mask Callback unite: NsiUsb_Tx_ApplyFcn(4);
      mask Display: image(imread('nsi.bmp'));text(0.5, 0.2, 'USB Tx', 'horizontalAlignment', 'center', 'verticalAlignment', 'base');plot([0.05 0.05 0.05 0.05 0.05 0.05 0.05 0.05 0.05 0.05]);port_label('input',1, 'rtd');
  UsbTx2 : S-Function  FunctionName=NsiUsb_Tx  Parameters=signame,resolution,offset,unite  SFunctionDeploymentMode=off  EnableBusSupport=off  mask(MUXlink Usb Tx){signame=x, resolution=1, offset=0, unite=km/h}
      mask prompts: signame "Signal name ?"; resolution "Resolution ?"; offset "Offset ?"; unite "Unit ?"
      mask help: Transmit a frame on the USB Channel.
      mask init:
      | NsiUsb_Tx_InitializationFcn();
      settings: OpenFcn=NsiUsb_Tx_OpenFcn();
      mask Help:
      | eval('block=get_param(gcb, ''RTWdata'');')
      | web([docroot '\toolbox\MUXlink\html\blocks/' block.MUXlink_BlockType '.html'])
      mask Callback signame: NsiUsb_Tx_ApplyFcn(1);
      mask Callback resolution: NsiUsb_Tx_ApplyFcn(2);
      mask Callback offset: NsiUsb_Tx_ApplyFcn(3);
      mask Callback unite: NsiUsb_Tx_ApplyFcn(4);
      mask Display: image(imread('nsi.bmp'));text(0.5, 0.2, 'USB Tx', 'horizontalAlignment', 'center', 'verticalAlignment', 'base');plot([0.05 0.05 0.05 0.05 0.05 0.05 0.05 0.05 0.05 0.05]);port_label('input',1, 'x');
  UsbTx3 : S-Function  FunctionName=NsiUsb_Tx  Parameters=signame,resolution,offset,unite  SFunctionDeploymentMode=off  EnableBusSupport=off  mask(MUXlink Usb Tx){signame=y, resolution=1, offset=0, unite=km/h}
      mask prompts: signame "Signal name ?"; resolution "Resolution ?"; offset "Offset ?"; unite "Unit ?"
      mask help: Transmit a frame on the USB Channel.
      mask init:
      | NsiUsb_Tx_InitializationFcn();
      settings: OpenFcn=NsiUsb_Tx_OpenFcn();
      mask Help:
      | eval('block=get_param(gcb, ''RTWdata'');')
      | web([docroot '\toolbox\MUXlink\html\blocks/' block.MUXlink_BlockType '.html'])
      mask Callback signame: NsiUsb_Tx_ApplyFcn(1);
      mask Callback resolution: NsiUsb_Tx_ApplyFcn(2);
      mask Callback offset: NsiUsb_Tx_ApplyFcn(3);
      mask Callback unite: NsiUsb_Tx_ApplyFcn(4);
      mask Display: image(imread('nsi.bmp'));text(0.5, 0.2, 'USB Tx', 'horizontalAlignment', 'center', 'verticalAlignment', 'base');plot([0.05 0.05 0.05 0.05 0.05 0.05 0.05 0.05 0.05 0.05]);port_label('input',1, 'y');
  UsbTx4 : S-Function  FunctionName=NsiUsb_Tx  Parameters=signame,resolution,offset,unite  SFunctionDeploymentMode=off  EnableBusSupport=off  mask(MUXlink Usb Tx){signame=z, resolution=1, offset=0, unite=km/h}
      mask prompts: signame "Signal name ?"; resolution "Resolution ?"; offset "Offset ?"; unite "Unit ?"
      mask help: Transmit a frame on the USB Channel.
      mask init:
      | NsiUsb_Tx_InitializationFcn();
      settings: OpenFcn=NsiUsb_Tx_OpenFcn();
      mask Help:
      | eval('block=get_param(gcb, ''RTWdata'');')
      | web([docroot '\toolbox\MUXlink\html\blocks/' block.MUXlink_BlockType '.html'])
      mask Callback signame: NsiUsb_Tx_ApplyFcn(1);
      mask Callback resolution: NsiUsb_Tx_ApplyFcn(2);
      mask Callback offset: NsiUsb_Tx_ApplyFcn(3);
      mask Callback unite: NsiUsb_Tx_ApplyFcn(4);
      mask Display: image(imread('nsi.bmp'));text(0.5, 0.2, 'USB Tx', 'horizontalAlignment', 'center', 'verticalAlignment', 'base');plot([0.05 0.05 0.05 0.05 0.05 0.05 0.05 0.05 0.05 0.05]);port_label('input',1, 'z');
  btnRTD_Input : Outport
  btnX_Input : Outport  Port=2
  btnY_Input : Outport  Port=3
  btnZ_Input : Outport  Port=4
  btnPumpFan_Input : Outport  Port=5
  btnAccyFan_Input : Outport  Port=6
  wires:
  DigitalInput2/1 -> UsbTx1/1, btnRTD_Input/1  "btnRTD_Input"
  DigitalInput4/1 -> UsbTx3/1, btnY_Input/1  "btnY_Input"
  DigitalInput3/1 -> UsbTx2/1, btnX_Input/1  "btnX_Input"
  DigitalInput1/1 -> UsbTx4/1, btnZ_Input/1  "btnZ_Input"
  DigitalInput5/1 -> btnPumpFan_Input/1  "btnPumpFan_Input"
  DigitalInput6/1 -> btnAccyFan_Input/1  "btnAccyFan_Input"
